simulink model "CarlaRosMatlab_VehicleControl"  (R2019b)
settings: Solver=FixedStepAuto  StartTime=0.0  StopTime=inf  FixedStep=0.2  RelTol=1e-3  EnableMultiTasking=on
model workspace (MAT data in the model file):
  SL_ROS_VariableLengthArrays_MaxSizes.CommonInfo.ArrayTruncateAction = 'EmitWarning'
  SL_ROS_VariableLengthArrays_MaxSizes.MsgTypeMap = containers.Map
  SL_ROS_VariableLengthArrays_MaxSizes.MsgTypeMap.serialization.keys = {'sensor_msgs/CompressedImage', 'sensor_msgs/Image', 'sensor_msgs/PointCloud2'}
  SL_ROS_VariableLengthArrays_MaxSizes.MsgTypeMap.serialization.values{1}(1).PropertyName = 'Format'
  SL_ROS_VariableLengthArrays_MaxSizes.MsgTypeMap.serialization.values{1}(1).DataType = 'uint8'
  SL_ROS_VariableLengthArrays_MaxSizes.MsgTypeMap.serialization.values{1}(1).MaxLength = 128
  SL_ROS_VariableLengthArrays_MaxSizes.MsgTypeMap.serialization.values{1}(2).PropertyName = 'Data'
  SL_ROS_VariableLengthArrays_MaxSizes.MsgTypeMap.serialization.values{1}(2).DataType = 'uint8'
  SL_ROS_VariableLengthArrays_MaxSizes.MsgTypeMap.serialization.values{1}(2).MaxLength = 128000
  SL_ROS_VariableLengthArrays_MaxSizes.MsgTypeMap.serialization.values{2}(1).PropertyName = 'Data'
  SL_ROS_VariableLengthArrays_MaxSizes.MsgTypeMap.serialization.values{2}(1).DataType = 'uint8'
  SL_ROS_VariableLengthArrays_MaxSizes.MsgTypeMap.serialization.values{2}(1).MaxLength = 3686400
  SL_ROS_VariableLengthArrays_MaxSizes.MsgTypeMap.serialization.values{2}(2).PropertyName = 'Encoding'
  SL_ROS_VariableLengthArrays_MaxSizes.MsgTypeMap.serialization.values{2}(2).DataType = 'uint8'
  SL_ROS_VariableLengthArrays_MaxSizes.MsgTypeMap.serialization.values{2}(2).MaxLength = 128
  SL_ROS_VariableLengthArrays_MaxSizes.MsgTypeMap.serialization.values{3}(1).PropertyName = 'Data'
  SL_ROS_VariableLengthArrays_MaxSizes.MsgTypeMap.serialization.values{3}(1).DataType = 'uint8'
  SL_ROS_VariableLengthArrays_MaxSizes.MsgTypeMap.serialization.values{3}(1).MaxLength = 179160
  SL_ROS_VariableLengthArrays_MaxSizes.MsgTypeMap.serialization.values{3}(2).PropertyName = 'Fields'
  SL_ROS_VariableLengthArrays_MaxSizes.MsgTypeMap.serialization.values{3}(2).DataType = 'sensor_msgs/PointField'
  SL_ROS_VariableLengthArrays_MaxSizes.MsgTypeMap.serialization.values{3}(2).MaxLength = 16
  SL_ROS_VariableLengthArrays_MaxSizes.MsgTypeMap.serialization.uniformity = 0
  SL_ROS_VariableLengthArrays_MaxSizes.MsgTypeMap.serialization.keyType = 'char'
  SL_ROS_VariableLengthArrays_MaxSizes.MsgTypeMap.serialization.valueType = 'any'
undefined symbols (not defined in the file): Brake, HandBrake, Reverse, Steer, Throttle
libraries: robotlib x13, visionsinks x4, visiontextngfix x2
settings Model: Creator=sprinkle  LastModifiedBy=aa
settings DataIOCC: ReturnWorkspaceOutputs=off
settings OptimizationCC: LifeSpan=Inf  MaxStackSize=64  EfficientTunableParamExpr=on
settings DebuggingCC: SFUnexpectedBacktrackingDiag=warning  SFNoUnconditionalDefaultTransitionDiag=warning  ArithmeticOperatorsInVariantConditions=warning
settings HardwareCC: ProdBitPerPointer=32  ProdBitPerSizeT=32  ProdBitPerPtrDiffT=32  ProdLargestAtomicFloat=None  ProdIntDivRoundTo=Undefined  ProdEndianess=Unspecified  ProdWordSize=32  ProdHWDeviceType=Generic->Unspecified (assume 32-bit Generic)
settings SFSimCC: SimUseLocalCustomCode=off  MATLABDynamicMemAlloc=off  CustomCodeUndefinedFunction=UseInterfaceOnly
settings RTWCC: SystemTargetFile=ert.tlc  HardwareBoard=Robot Operating System (ROS)  TLCOptions=-aInlineSetEventsForThisBaseRateFcn=TLC_FALSE -aSuppressMultiTaskScheduler=TLC_FALSE -aRateBasedStepFcn=0  TemplateMakefile=ert_default_tmf  GenerateReport=on  RTWUseLocalCustomCode=off  Toolchain=Catkin  IncludeHyperlinkInReport=on  LaunchReport=on  TargetLang=C++  GenerateTraceInfo=on  GenerateTraceReport=on  GenerateTraceReportSl=on  GenerateTraceReportSf=on  GenerateTraceReportEml=on
settings CodeAppCC: ForceParamTrailComments=on  IgnoreCustomStorageClasses=off  OperatorAnnotations=on  SimulinkDataObjDesc=on  SFDataObjDesc=on  MATLABFcnDesc=on  InsertBlockDesc=on  StateflowObjectComments=on  MATLABSourceComments=on
settings ERTTargetCC: MultiwordLength=2048
settings ConfigComp: CovMetricSettings=dw  CovHtmlReporting=on  CovSaveCumulativeToWorkspaceVar=on  CovSaveSingleToWorkspaceVar=on  CovExternalEMLEnable=off

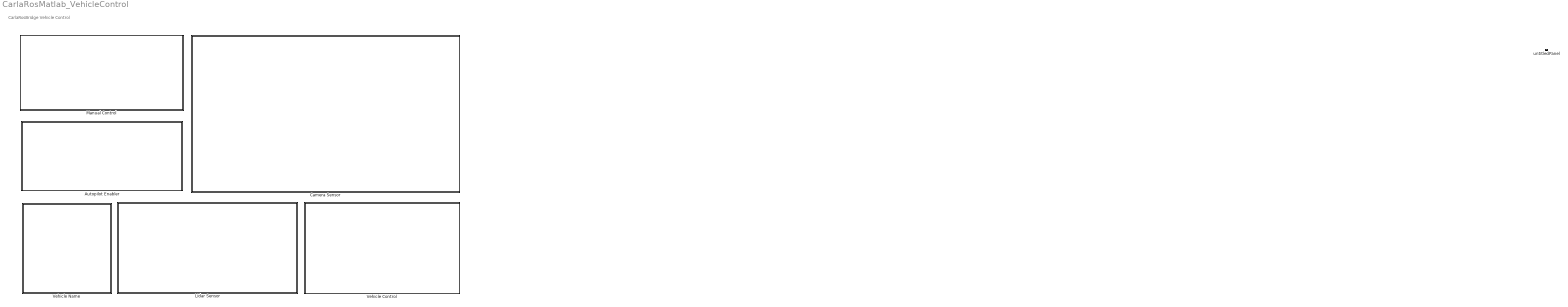
== system CarlaRosMatlab_VehicleControl ==
  note: CarlaRosBridge Vehicle Control
  Autopilot Enabler : Subsystem
  Camera Sensor : Subsystem
  Lidar Sensor : Subsystem
  Manual Control : Subsystem
  Vehicle Control : Subsystem
  Vehicle Name : Subsystem
  untitledPanel : Subsystem  Tag=HiddenForWebPanel  IsWebBlockPanel=on

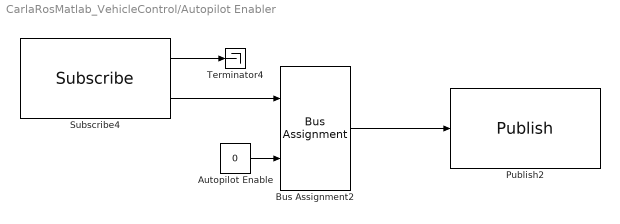
== system CarlaRosMatlab_VehicleControl/Autopilot Enabler ==
  Autopilot Enable : Constant  Value=0  OutDataTypeStr=boolean
  Bus Assignment2 : BusAssignment  AssignedSignals=Data
  Publish2 : robotlib/Publish  topicSource=Select from ROS network  topic=/carla/ego_vehicle/enable_autopilot  messageType=std_msgs/Bool  messageQueueLength=1
      settings: SourceProductName=ROS Toolbox
  Subscribe4 : robotlib/Subscribe  topicSource=Select from ROS network  topic=/carla/ego_vehicle/enable_autopilot  messageType=std_msgs/Bool  sampleTime=-1  messageQueueLength=1
      settings: SourceProductName=ROS Toolbox
  Terminator4 : Terminator
  wires:
  Subscribe4/1 -> Terminator4/1
  Subscribe4/2 -> Bus Assignment2/1
  Bus Assignment2/1 -> Publish2/1
  Autopilot Enable/1 -> Bus Assignment2/2

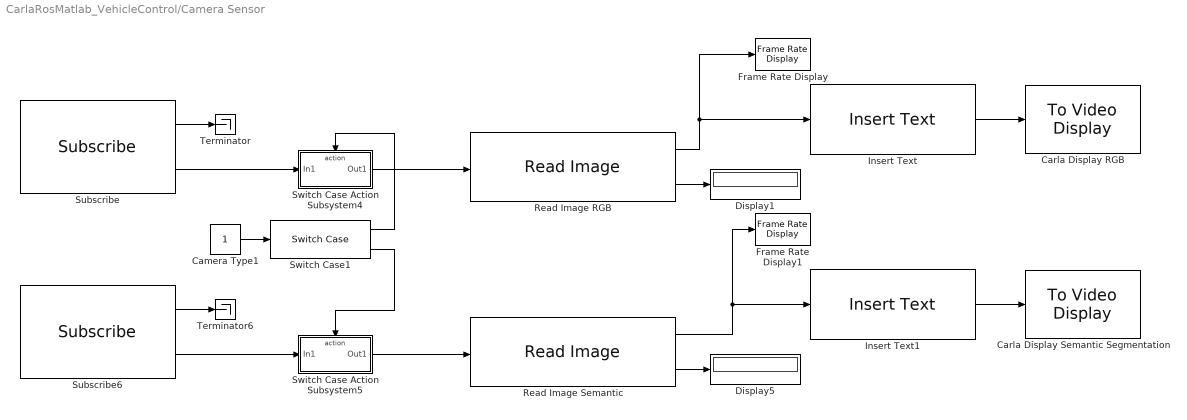
== system CarlaRosMatlab_VehicleControl/Camera Sensor ==
  Camera Type1 : Constant
  Carla Display RGB : visionsinks/To Video Display  windowSizeMode=Normal  openAtMdlStart=on  fullScreen=off  videoWindowX=527  videoWindowY=24  saveWindowSize=off  videoWindowWidth=551  videoWindowHeight=468  inputColorFormat=RGB  inputType=Obsolete  imagePorts=One multidimensional signal  OutputDevice=On-screen video monitor  dataOrg=Column-major  isWindowOpen=off
      settings: SourceProductName=Computer Vision Toolbox
  Carla Display Semantic Segmentation : visionsinks/To Video Display  windowSizeMode=Normal  openAtMdlStart=on  fullScreen=off  videoWindowX=65  videoWindowY=415  saveWindowSize=off  videoWindowWidth=950  videoWindowHeight=769  inputColorFormat=RGB  inputType=Obsolete  imagePorts=One multidimensional signal  OutputDevice=On-screen video monitor  dataOrg=Column-major  isWindowOpen=off
      settings: SourceProductName=Computer Vision Toolbox
  Display1 : Display
  Display5 : Display
  Frame Rate Display : visionsinks/Frame Rate Display  UpdateRate=10
      settings: SourceProductName=Computer Vision Toolbox  SourceProductBaseCode=VP
  Frame Rate Display1 : visionsinks/Frame Rate Display  UpdateRate=10
      settings: SourceProductName=Computer Vision Toolbox  SourceProductBaseCode=VP
  Insert Text : visiontextngfix/Insert Text  inputType=Obsolete  theText='Carla Ros Bridge RGB Camera'  getTextLocFrom=Specify via dialog  textLoc=[1 1]  getTextColorFrom=Specify via dialog  textColor=[0 0 0]  getTextIntensityFrom=Specify via dialog  textIntensity=0  getTextOpacityFrom=Specify via dialog  textOpacity=1.0  dummyVar2=0  dummyVar3=0  dummyVar4=0  imagePorts=One multidimensional signal  isInputTransposed=off  fontFace=LucidaSansRegular  dummyVar1=0  blockFontSize=24  antiAliased=on
      settings: SourceProductName=Computer Vision Toolbox  SourceProductBaseCode=VP
  Insert Text1 : visiontextngfix/Insert Text  inputType=Obsolete  theText='Carla Ros Bridge Semantic Segmentation'  getTextLocFrom=Specify via dialog  textLoc=[1 1]  getTextColorFrom=Specify via dialog  textColor=[0 0 0]  getTextIntensityFrom=Specify via dialog  textIntensity=0  getTextOpacityFrom=Specify via dialog  textOpacity=1.0  dummyVar2=0  dummyVar3=0  dummyVar4=0  imagePorts=One multidimensional signal  isInputTransposed=off  fontFace=LucidaSansRegular  dummyVar1=0  blockFontSize=24  antiAliased=on
      settings: SourceProductName=Computer Vision Toolbox  SourceProductBaseCode=VP
  Read Image RGB : robotlib/Read Image  MaximumImageSize=[600, 800]  ImageEncoding=bgra8  ShowAlphaOutput=off  ShowErrorCodeOutput=on  VariableSizeOutputs=on
      settings: SourceProductName=Robotics System Toolbox  SourceProductBaseCode=RO
  Read Image Semantic : robotlib/Read Image  MaximumImageSize=[540, 960]  ImageEncoding=bgra8  ShowAlphaOutput=off  ShowErrorCodeOutput=on  VariableSizeOutputs=on
      settings: SourceProductName=Robotics System Toolbox  SourceProductBaseCode=RO
  Subscribe : robotlib/Subscribe  topicSource=Select from ROS network  topic=/carla/ego_vehicle/camera/rgb/front/image_color  messageType=sensor_msgs/Image  sampleTime=-1  messageQueueLength=1
      settings: SourceProductBaseCode=RO
  Subscribe6 : robotlib/Subscribe  topicSource=Select from ROS network  topic=/carla/ego_vehicle/camera/semantic_segmentation/fronts/image_segmentation  messageType=sensor_msgs/Image  sampleTime=-1  messageQueueLength=1
      settings: SourceProductBaseCode=RO
  Switch Case Action Subsystem4 : Subsystem  TreatAsAtomicUnit=on
  Switch Case Action Subsystem5 : Subsystem  TreatAsAtomicUnit=on
  Switch Case1 : SwitchCase  CaseConditions={0,1}  ShowDefaultCase=off
  Terminator : Terminator
  Terminator6 : Terminator
  wires:
  Subscribe6/1 -> Terminator6/1
  Insert Text1/1 -> Carla Display Semantic Segmentation/1
  Switch Case1/2 -> Switch Case Action Subsystem5/Action
  Subscribe/2 -> Switch Case Action Subsystem4/1(In1)
  Read Image Semantic/1 -> Insert Text1/1, Frame Rate Display1/1
  Switch Case Action Subsystem4/1(Out1) -> Read Image RGB/1
  Read Image RGB/1 -> Frame Rate Display/1, Insert Text/1
  Read Image Semantic/2 -> Display5/1
  Subscribe6/2 -> Switch Case Action Subsystem5/1(In1)
  Switch Case1/1 -> Switch Case Action Subsystem4/Action
  Subscribe/1 -> Terminator/1
  Read Image RGB/2 -> Display1/1
  Switch Case Action Subsystem5/1(Out1) -> Read Image Semantic/1
  Camera Type1/1 -> Switch Case1/1
  Insert Text/1 -> Carla Display RGB/1

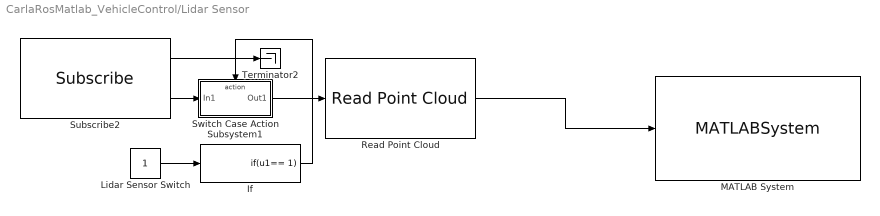
== system CarlaRosMatlab_VehicleControl/Lidar Sensor ==
  If : If  IfExpression=u1== 1  ShowElse=off
  Lidar Sensor Switch : Constant
  MATLAB System : MATLABSystem  System=viewPC  SimulateUsing=Interpreted execution
      mask Type: viewPC
      mask Display:
      | disp('viewPC');
      | port_label('input',1,'xyzpoint');
  Read Point Cloud : robotlib/Read Point Cloud  MaximumPointCloudSize=[1, 14273]  PreserveStructure=off  ShowRGBOutput=off  ShowIntensityOutput=off  ShowErrorCodeOutput=off  VariableSizeOutputs=off
      settings: SourceProductName=ROS Toolbox  SourceProductBaseCode=RR
  Subscribe2 : robotlib/Subscribe  topicSource=Select from ROS network  topic=/carla/ego_vehicle/lidar/lidar1/point_cloud  messageType=sensor_msgs/PointCloud2  sampleTime=-1  messageQueueLength=1
      settings: SourceProductName=ROS Toolbox
  Switch Case Action Subsystem1 : Subsystem  TreatAsAtomicUnit=on
  Terminator2 : Terminator
  wires:
  Switch Case Action Subsystem1/1(Out1) -> Read Point Cloud/1
  If/1 -> Switch Case Action Subsystem1/Action
  Subscribe2/1 -> Terminator2/1
  Read Point Cloud/1 -> MATLAB System/1
  Lidar Sensor Switch/1 -> If/1
  Subscribe2/2 -> Switch Case Action Subsystem1/1(In1)

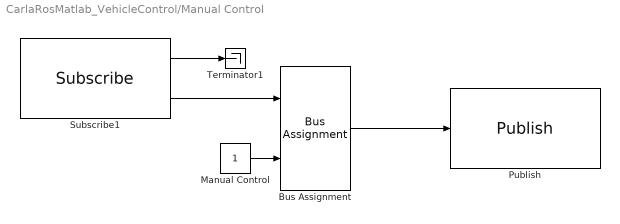
== system CarlaRosMatlab_VehicleControl/Manual Control ==
  Bus Assignment : BusAssignment  AssignedSignals=Data
  Manual Control : Constant  OutDataTypeStr=boolean
  Publish : robotlib/Publish  topicSource=Select from ROS network  topic=/carla/ego_vehicle/vehicle_control_manual_override  messageType=std_msgs/Bool  messageQueueLength=1
      settings: SourceProductName=ROS Toolbox
  Subscribe1 : robotlib/Subscribe  topicSource=Select from ROS network  topic=/carla/ego_vehicle/vehicle_control_manual_override  messageType=std_msgs/Bool  sampleTime=-1  messageQueueLength=1
      settings: SourceProductName=ROS Toolbox
  Terminator1 : Terminator
  wires:
  Subscribe1/2 -> Bus Assignment/1
  Manual Control/1 -> Bus Assignment/2
  Bus Assignment/1 -> Publish/1
  Subscribe1/1 -> Terminator1/1

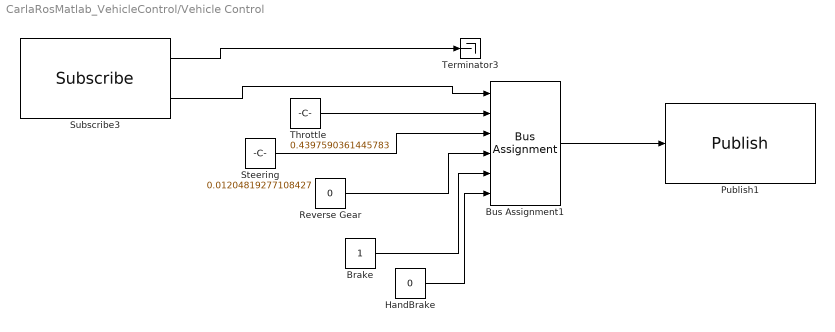
== system CarlaRosMatlab_VehicleControl/Vehicle Control ==
  Brake : Constant  OutDataTypeStr=single
  Bus Assignment1 : BusAssignment  AssignedSignals=Throttle,Steer,Reverse,Brake,HandBrake
  HandBrake : Constant  Value=0  OutDataTypeStr=boolean
  Publish1 : robotlib/Publish  topicSource=Select from ROS network  topic=/carla/ego_vehicle/vehicle_control_cmd_manual  messageType=carla_msgs/CarlaEgoVehicleControl  messageQueueLength=1
      settings: SourceProductName=ROS Toolbox
  Reverse Gear : Constant  Value=0  OutDataTypeStr=boolean
  Steering : Constant  Value=0.01204819277108427  OutDataTypeStr=single
  Subscribe3 : robotlib/Subscribe  topicSource=Select from ROS network  topic=/carla/ego_vehicle/vehicle_control_cmd_manual  messageType=carla_msgs/CarlaEgoVehicleControl  sampleTime=-1  messageQueueLength=1
      settings: SourceProductName=ROS Toolbox
  Terminator3 : Terminator
  Throttle : Constant  Value=0.4397590361445783  OutDataTypeStr=single
  wires:
  HandBrake/1 -> Bus Assignment1/6
  Steering/1 -> Bus Assignment1/3
  Bus Assignment1/1 -> Publish1/1
  Throttle/1 -> Bus Assignment1/2
  Brake/1 -> Bus Assignment1/5
  Subscribe3/2 -> Bus Assignment1/1
  Subscribe3/1 -> Terminator3/1
  Reverse Gear/1 -> Bus Assignment1/4

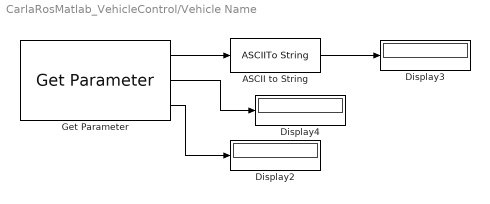
== system CarlaRosMatlab_VehicleControl/Vehicle Name ==
  ASCII to String : ASCIIToString
  Display2 : Display
  Display3 : Display
  Display4 : Display
  Get Parameter : robotlib/Get Parameter  ParameterSource=Select from ROS network  ParameterName=/carla_ego_vehicle_ego_vehicle/role_name  ParameterType=uint8[] (string)  ParameterMaxArrayLength=16  ParameterInitialValue=0.0  SampleTime=-1  ShowErrorCodeOutput=on  ModelName=CarlaRosMatlab_Updated  BlockId=ParamGet_CarlaRosMatlab_Updated_212
      settings: SourceProductName=ROS Toolbox  SourceProductBaseCode=RR
  wires:
  Get Parameter/1 -> ASCII to String/1
  Get Parameter/3 -> Display2/1
  Get Parameter/2 -> Display4/1
  ASCII to String/1 -> Display3/1

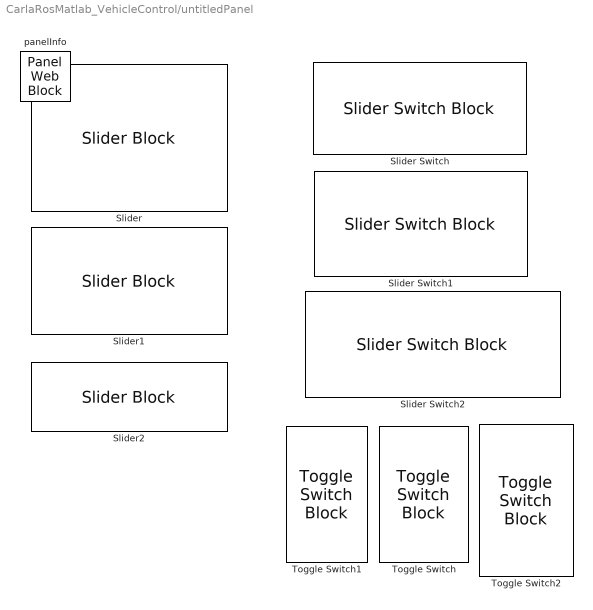
== system CarlaRosMatlab_VehicleControl/untitledPanel ==
  Slider : SliderBlock  Tag=HiddenForWebPanel  PanelInfo="{\"panelId\":\"panelId-a6fc69b6-b572-4193-922b-c04a305ae533\",\"type\":\"panelChild\",\"version\":\"2019b\",\"zIndex\":1500005}"  ScaleMax=1
  Slider Switch : SliderSwitchBlock  Tag=HiddenForWebPanel  PanelInfo="{\"panelId\":\"panelId-a6fc69b6-b572-4193-922b-c04a305ae533\",\"type\":\"panelChild\",\"version\":\"2019b\",\"zIndex\":1500002}"
      settings: Values={{'Off', 'On'}, [0 1]}
  Slider Switch1 : SliderSwitchBlock  Tag=HiddenForWebPanel  PanelInfo="{\"panelId\":\"panelId-a6fc69b6-b572-4193-922b-c04a305ae533\",\"type\":\"panelChild\",\"version\":\"2019b\",\"zIndex\":1500004}"
      settings: Values={{'Off', 'On'}, [0 1]}
  Slider Switch2 : SliderSwitchBlock  Tag=HiddenForWebPanel  PanelInfo="{\"panelId\":\"panelId-a6fc69b6-b572-4193-922b-c04a305ae533\",\"type\":\"panelChild\",\"version\":\"2019b\",\"zIndex\":1500009}"
      settings: Values={{'RGB', 'Semantic Segmentation'}, [0 1]}
  Slider1 : SliderBlock  Tag=HiddenForWebPanel  PanelInfo="{\"panelId\":\"panelId-a6fc69b6-b572-4193-922b-c04a305ae533\",\"type\":\"panelChild\",\"version\":\"2019b\",\"zIndex\":1500007}"  ScaleMin=-1  ScaleMax=1
  Slider2 : SliderBlock  Tag=HiddenForWebPanel  PanelInfo="{\"panelId\":\"panelId-a6fc69b6-b572-4193-922b-c04a305ae533\",\"type\":\"panelChild\",\"version\":\"2019b\",\"zIndex\":1500003}"  ScaleMax=1
  Toggle Switch : ToggleSwitchBlock  Tag=HiddenForWebPanel  PanelInfo="{\"panelId\":\"panelId-a6fc69b6-b572-4193-922b-c04a305ae533\",\"type\":\"panelChild\",\"version\":\"2019b\",\"zIndex\":1500006}"
      settings: Values={{'Off', 'On'}, [0 1]}
  Toggle Switch1 : ToggleSwitchBlock  Tag=HiddenForWebPanel  PanelInfo="{\"panelId\":\"panelId-a6fc69b6-b572-4193-922b-c04a305ae533\",\"type\":\"panelChild\",\"version\":\"2019b\",\"zIndex\":1500001}"
      settings: Values={{'Off', 'On'}, [0 1]}
  Toggle Switch2 : ToggleSwitchBlock  Tag=HiddenForWebPanel  PanelInfo="{\"panelId\":\"panelId-a6fc69b6-b572-4193-922b-c04a305ae533\",\"type\":\"panelChild\",\"version\":\"2019b\",\"zIndex\":1500008}"
      settings: Values={{'Off', 'On'}, [0 1]}
  panelInfo : PanelWebBlock  Tag=HiddenForWebPanel  PanelInfo="{\"compacted\":false,\"height\":570,\"left\":98,\"panelId\":\"panelId-a6fc69b6-b572-4193-922b-c04a305ae533\",\"top\":143,\"type\":\"panel\",\"version\":\"2019b\",\"visible\":true,\"width\":622,\"zIndex\":1500001}"  PanelSnapshot=<binary blob, 61680 chars, not shown>

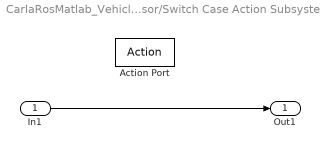
== system CarlaRosMatlab_VehicleControl/Camera Sensor/Switch Case Action Subsystem4 ==
  In1 : Inport
  Action Port : ActionPort  ActionPortLabel=case [ 0 ]:
  Out1 : Outport
  wires:
  In1/1 -> Out1/1

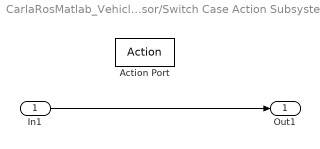
== system CarlaRosMatlab_VehicleControl/Camera Sensor/Switch Case Action Subsystem5 ==
  In1 : Inport
  Action Port : ActionPort  ActionPortLabel=case [ 1 ]:
  Out1 : Outport
  wires:
  In1/1 -> Out1/1

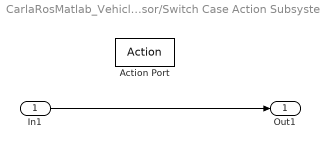
== system CarlaRosMatlab_VehicleControl/Lidar Sensor/Switch Case Action Subsystem1 ==
  In1 : Inport
  Action Port : ActionPort  ActionPortLabel=if(u1== 1)
  Out1 : Outport
  wires:
  In1/1 -> Out1/1
